simulink model "Syn_Leader_Follower_ext1"  (R2021a)
settings: Solver=VariableStepAuto  StartTime=0.0  StopTime=2  RelTol=1e-3
settings Model: Creator=JianFongLee  LastModifiedBy=JianFongLee

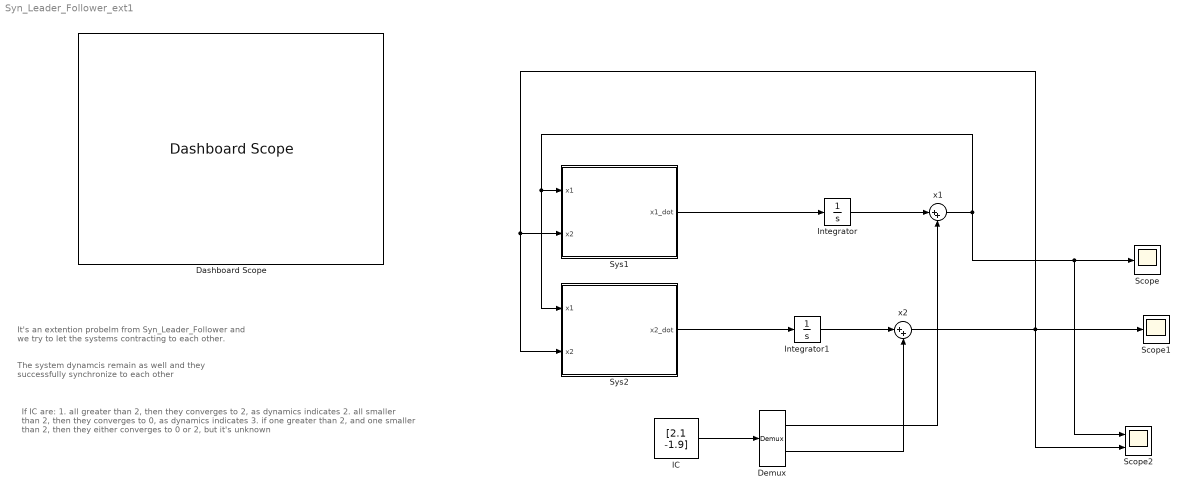
== system Syn_Leader_Follower_ext1 ==
  note: If IC are:
      | 1.	all greater than 2, then they converges to 2, as dynamics indicates
      | 2.	all smaller than 2, then they converges to 0, as dynamics indicates
      | 3.	if one greater than 2, and one smaller than 2, then they either converges to 0 or 2, 		but it's unknown
  note: The system dynamcis remain as well
      | and they successfully synchronize to each other
  note: It's an extention probelm from Syn_Leader_Follower
      | and we try to let the systems contracting to each other.
  Dashboard Scope : DashboardScope
  Demux : Demux  Outputs=2
      settings: DisplayOption=none
  IC : Constant  Value=[2.1 -1.9]
  Integrator : Integrator
  Integrator1 : Integrator
  Scope : Scope
  Scope1 : Scope
  Scope2 : Scope  NumInputPorts=2
  Sys1 : MATLAB Function  TreatAsAtomicUnit=on
  Sys2 : MATLAB Function  TreatAsAtomicUnit=on
  x1 : Sum  Inputs=|++
  x2 : Sum  Inputs=|++
  wires:
  Sys1/1(x1_dot) -> Integrator/1
  Integrator/1 -> x1/1
  x1/1 -> Scope2/1, Scope/1, Sys2/1(x1), Sys1/1(x1)
  Sys2/1(x2_dot) -> Integrator1/1
  IC/1 -> Demux/1
  Demux/1 -> x1/2
  Integrator1/1 -> x2/1
  Demux/2 -> x2/2
  x2/1 -> Scope2/2, Scope1/1, Sys1/2(x2), Sys2/2(x2)

== matlab function Syn_Leader_Follower_ext1/Sys1 ==
  data: x1 input; x1_dot output; x2 input
function x1_dot = fcn(x1,x2)
%%% System 1
u = -2*(x1^2 - x2^2);

x1_dot = -x1*(x1-2)*(x1-2) + u;

end

== matlab function Syn_Leader_Follower_ext1/Sys2 ==
  data: x1 input; x2_dot output; x2 input
function x2_dot = fcn(x1,x2)
 
%%% System 2
u = 4*(x1^2 - x2^2);
x2_dot = -x2*(x2-2)*(x2-2) + u;

end
